simulink model "tx_host"  (R2016a)
settings: Solver=ode4  StartTime=0.0  StopTime=inf  FixedStep=0.001  RelTol=1e-3
libraries: xpcutilitieslib x1, xpcrtudplib x1, instrumentlib x1
settings Model: xpc_rtwmakecfg_data=_xpcnblib__xpcetherlib__xpcether8255xlib__xpcetherGbElib__xpciplib_  Creator=Biorobotics  LastModifiedBy=Biorobotics
settings SolverCC: EnableConcurrentExecution=on  ConcurrentTasks=on  PositivePriorityOrder=on  AutoInsertRateTranBlk=on
settings DataIOCC: SaveFormat=StructureWithTime
settings OptimizationCC: BlockReduction=off  OptimizeBlockIOStorage=off  BufferReuse=off  GlobalBufferReuse=off  ExpressionFolding=off  LocalBlockOutputs=off
settings HardwareCC: ProdBitPerPointer=32  ProdLargestAtomicFloat=None  ProdWordSize=32  ProdLongLongMode=on  ProdHWDeviceType=Generic->32-bit x86 compatible
settings RTWCC: SystemTargetFile=slrt.tlc  TemplateMakefile=slrt_default_tmf  Description=Simulink Real-Time  RTWCompilerOptimization=on

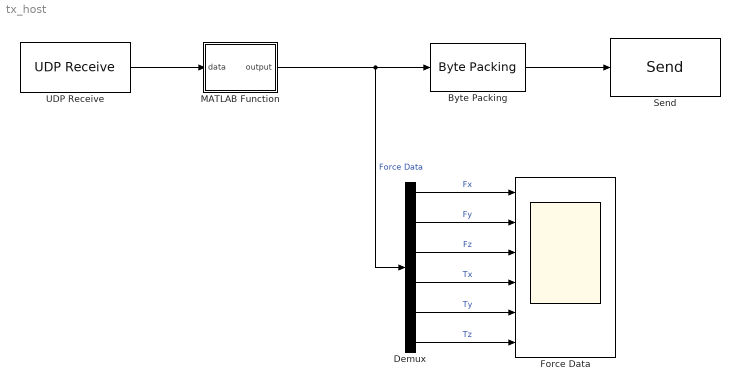
== system tx_host ==
  "Byte Packing " : xpcutilitieslib/Byte Packing   MaskPackedDataType=uint8  MaskUnpackedDataTypes={'double'}  MaskAlignment=1
  Demux : Demux  Outputs=6
  Force Data : Scope  NumInputPorts=6
  MATLAB Function : MATLAB Function  TreatAsAtomicUnit=on
  "Send " : xpcrtudplib/Legacy UDP/Send   ipAddress=192.168.1.3  ipPort=25000  localPort=-1  vblLen=off  sampletime=0.001
  UDP Receive : instrumentlib/UDP Receive  Host=192.168.1.1  Port=49152  LocalPort=54546  DataSize=36  EnableBlockingMode=on  Timeout=1  SampleTime=0.001  DataType=uint8  ByteOrder=BigEndian
  wires:
  "Byte Packing "/1 -> "Send "/1
  UDP Receive/1 -> MATLAB Function/1(data)
  MATLAB Function/1(output) -> Demux/1, "Byte Packing "/1  "Force Data"
  Demux/1 -> Force Data/1  "Fx"
  Demux/2 -> Force Data/2  "Fy"
  Demux/3 -> Force Data/3  "Fz"
  Demux/4 -> Force Data/4  "Tx"
  Demux/5 -> Force Data/5  "Ty"
  Demux/6 -> Force Data/6  "Tz"

== matlab function tx_host/MATLAB Function ==
  data: data input; output output
function output = fcn(data)
%#codegen
NUM_RDT_FIELDS = 9;
    calmat=[1 1 1 25 25 35 250 250 250];
    RDTPacket = zeros(1,NUM_RDT_FIELDS, 'int32');

    for i = NUM_RDT_FIELDS:-1:1
        %display(data(i*4));
        %display(int32(data(i*4)));
        index = (i-1)*4 + 1;
        RDTPacket(i) = bitand(int32(data(index)), hex2dec('ff'));
        j = (i-1)*4 + 2;
        while j < ((i-1)*4 + 5)
            shiftedPacket = bitshift(RDTPacket(i), 8);
            RDTPacket(i) = bitor(shiftedPacket, bitand(int32(data(j)), ...
                hex2dec('ff')));
            j = j + 1;
        end
    end
    y=double(RDTPacket)./(1e6.*calmat);
    output=y(4:9);
end
